simulink model "SimModeleLineaire"  (R2018b)
settings: Solver=VariableStepAuto  StartTime=0.0  StopTime=1  RelTol=1e-3
values from neighbouring files (symbols this model uses):
  A = double(subs(A))    [ModeleLineaire.m]    (also in Projet_S5_lin.m = double(A))
  B = double(subs(B))    [ModeleLineaire.m]    (also in Projet_S5_lin.m = double(B))
  C = double(subs(C))    [ModeleLineaire.m]    (also in Projet_S5_lin.m = double(C))
  D = [mat_Zero73]    [ModeleLineaire.m]    (also in Projet_S5_lin.m = double(D))
settings Model: Creator=Vincent  LastModifiedBy=Vincent

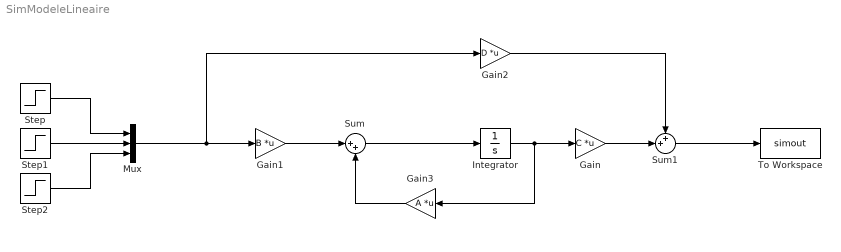
== system SimModeleLineaire ==
  Gain : Gain  Gain=C  Multiplication=Matrix(K*u)
  Gain1 : Gain  Gain=B  Multiplication=Matrix(K*u)
  Gain2 : Gain  Gain=D  Multiplication=Matrix(K*u)
  Gain3 : Gain  Gain=A  Multiplication=Matrix(K*u)
  Integrator : Integrator
  Mux : Mux  Inputs=3
  Step : Step  SampleTime=0
  Step1 : Step  SampleTime=0
  Step2 : Step  SampleTime=0
  Sum : Sum  Inputs=|++
  Sum1 : Sum  Inputs=++|
  To Workspace : ToWorkspace  VariableName=simout  SaveFormat=Timeseries  SampleTime=-1
  wires:
  Integrator/1 -> Gain3/1, Gain/1
  Gain3/1 -> Sum/2
  Gain/1 -> Sum1/2
  Gain2/1 -> Sum1/1
  Mux/1 -> Gain2/1, Gain1/1
  Sum1/1 -> To Workspace/1
  Step/1 -> Mux/1
  Step2/1 -> Mux/3
  Step1/1 -> Mux/2
  Gain1/1 -> Sum/1
  Sum/1 -> Integrator/1
